simulink model "Base_Map_cs"  (R2019a)
settings: Solver=FixedStepDiscrete  StartTime=0.0  StopTime=15  FixedStep=1/300  RelTol=1e-3
PreLoadFcn:
  | mbxruntime.callbacks.PreLoadFcn(bdroot);
  | check_NUTS_defined
  | model_closed = 0;
  | assignin('base',['model_closed_' bdroot],false);
PostLoadFcn:
  | mbxruntime.callbacks.PostLoadFcn(bdroot);
InitFcn:
  | mbxruntime.callbacks.InitFcn(bdroot);
StartFcn:
  | mbxruntime.callbacks.StartFcn(bdroot);
StopFcn:
  | mbxruntime.callbacks.StopFcn(bdroot);;
  | 
model workspace: external: MAT-File .\Base_Map_S_cs_hws.mat (data not in the file)
undefined symbols (not defined in the file or in its folder): AngularVelocity, Clock_, Data, Data_SL_Info, DiscIntNeverNeededParam, Encoding, Encoding_SL_Info, Header, Height, InitImageOutputDir, LinearAcceleration, mbxruntime, Orientation, Pose, Poses, Poses_SL_Info, Position, Step, tabledata, Twist, Width
libraries: PBCSimulinkLibrary x53, robotlib x26, simulink_extras x19, PreScanSimulinkLibrary x6, dspindex x4, robotcorelib x2, sharedtransform x2, visionconversions x1, visionsinks x1
(part 5 of 8)

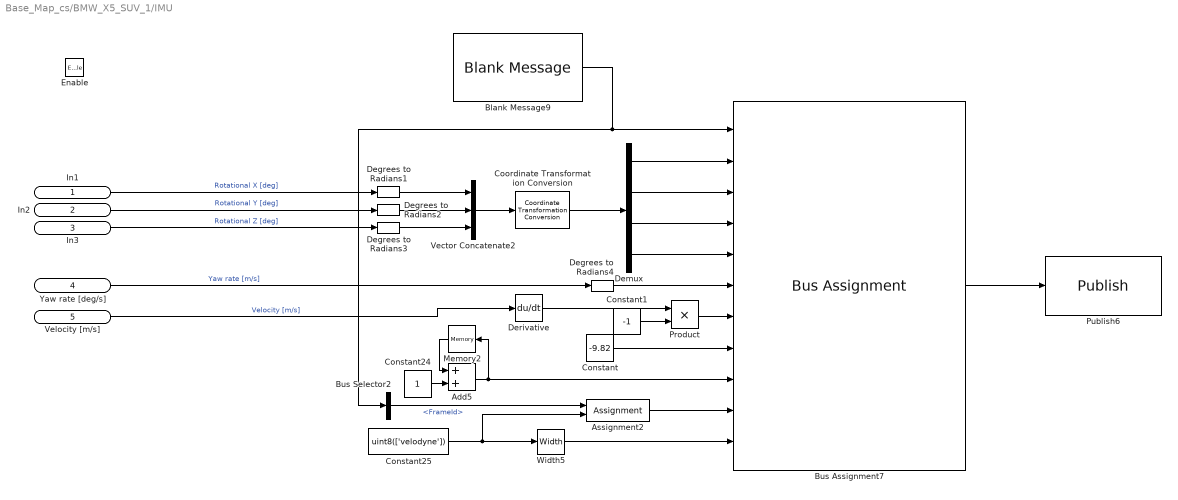
== system Base_Map_cs/BMW_X5_SUV_1/IMU ==
  In1 : Inport
  In2 : Inport  Port=2
  In3 : Inport  Port=3
  Yaw rate [deg/s] : Inport  Port=4
  Velocity [m/s] : Inport  Port=5
  Enable : EnablePort
  Add5 : Sum
  Assignment2 : Assignment  OutputInitialize=Specify size for each dimension in table  DiagnosticForDimensions=Warning  IndexOptions=Starting index (dialog)  Indices=1  OutputSizes=1000
  Blank Message9 : robotlib/Blank Message  messageClass=Message  entityType=sensor_msgs/Imu  messageType=sensor_msgs/Imu  SampleTime=inf
      settings: SourceProductBaseCode=RO
  Bus Assignment7 : BusAssignment  AssignedSignals=Orientation.W,Orientation.X,Orientation.Y,Orientation.Z,AngularVelocity.Z,LinearAcceleration.X,LinearAcceleration.Z,Header.Seq,Header.FrameId,Header.FrameId_SL_Info.CurrentLength
  Bus Selector2 : BusSelector  OutputSignals=Header.FrameId
  Constant : Constant  Value=-9.82
  Constant1 : Constant  Value=-1
  Constant24 : Constant  OutDataTypeStr=uint32
  Constant25 : Constant  Value=uint8(['velodyne'])
  Coordinate Transformation Conversion : robotcorelib/Coordinate Transformation Conversion  InputRepresentation=Euler Angles  InputEulerSequence=XYZ  ShowTrVecInputPort=on  OutputRepresentation=Quaternion  OutputEulerSequence=ZYX  ShowTrVecOutputPort=on  SimulateUsing=Interpreted execution
      settings: SourceProductBaseCode=RO
  Degrees to Radians{1..4} (4 alike) : simulink_extras/Transformations/Degrees to Radians
  Demux : Demux
  Derivative : Derivative
  Memory2 : Memory  InheritSampleTime=on
  Product : Product
  Publish6 : robotlib/Publish  topicSource=Select from ROS network  topic=/imu_raw  messageType=sensor_msgs/Imu  messageQueueLength=1
      settings: SourceProductBaseCode=RO
  Vector Concatenate2 : Concatenate  NumInputs=3
  Width5 : Width  DataType=uint32
  wires:
  Product/1 -> Bus Assignment7/7
  Constant1/1 -> Product/2
  In3/1 -> Degrees to Radians3/1  "Rotational Z [deg]"
  In2/1 -> Degrees to Radians2/1  "Rotational Y [deg]"
  In1/1 -> Degrees to Radians1/1  "Rotational X [deg]"
  Constant/1 -> Bus Assignment7/8
  Velocity [m/s]/1 -> Derivative/1  "Velocity [m/s]"
  Yaw rate [deg/s]/1 -> Degrees to Radians4/1  "Yaw rate [m/s]"
  Demux/4 -> Bus Assignment7/5
  Demux/1 -> Bus Assignment7/2
  Coordinate Transformation Conversion/1 -> Demux/1
  Demux/3 -> Bus Assignment7/4
  Vector Concatenate2/1 -> Coordinate Transformation Conversion/1
  Degrees to Radians3/1 -> Vector Concatenate2/3
  Demux/2 -> Bus Assignment7/3
  Degrees to Radians2/1 -> Vector Concatenate2/2
  Derivative/1 -> Product/1
  Assignment2/1 -> Bus Assignment7/10
  Degrees to Radians4/1 -> Bus Assignment7/6
  Memory2/1 -> Add5/1
  Bus Assignment7/1 -> Publish6/1
  Add5/1 -> Bus Assignment7/9, Memory2/1
  Width5/1 -> Bus Assignment7/11
  Blank Message9/1 -> Bus Assignment7/1, Bus Selector2/1
  Bus Selector2/1 -> Assignment2/1  "<FrameId>"
  Constant25/1 -> Width5/1, Assignment2/2
  Constant24/1 -> Add5/2
  Degrees to Radians1/1 -> Vector Concatenate2/1

== system Base_Map_cs/BMW_X5_SUV_1/PhysicsBasedCameraSensor_1_PBCPose_Control_Mux ==
  Position [m] : Inport
  Orientation [rad] : Inport  Port=2
  Bus Creator1 : BusCreator  Inputs=12  OutDataTypeStr=Bus: PRESCAN_PBCPOSE_DATA  NonVirtualBus=on
  Demux{,1..3} (4 alike) : Demux  Outputs=3
  SignalChanged : PBCSimulinkLibrary/SignalChanged  SystemSampleTime=-1
  SignalChanged1 : PBCSimulinkLibrary/SignalChanged  SystemSampleTime=-1
  Bus : Outport
  wires:
  Demux1/3 -> Bus Creator1/12  "OrientationYaw"
  Demux1/2 -> Bus Creator1/11  "OrientationPitch"
  Demux1/1 -> Bus Creator1/10  "OrientationRoll"
  Demux3/3 -> Bus Creator1/9  "OrientationYawDefined"
  Demux3/2 -> Bus Creator1/8  "OrientationPitchDefined"
  Demux3/1 -> Bus Creator1/7  "OrientationRollDefined"
  Demux/3 -> Bus Creator1/6  "PositionZ"
  Demux/2 -> Bus Creator1/5  "PositionY"
  Demux/1 -> Bus Creator1/4  "PositionX"
  Demux2/3 -> Bus Creator1/3  "PositionZDefined"
  Demux2/2 -> Bus Creator1/2  "PositionYDefined"
  Demux2/1 -> Bus Creator1/1  "PositionXDefined"
  SignalChanged1/1 -> Demux3/1
  SignalChanged/1 -> Demux2/1
  Bus Creator1/1 -> Bus/1
  Position [m]/1 -> SignalChanged/1, Demux/1
  Orientation [rad]/1 -> SignalChanged1/1, Demux1/1

== system Base_Map_cs/BMW_X5_SUV_1/PhysicsBasedCameraSensor_1_PBC_Control_Mux ==
  IntegrationTime [s] : Inport
  DigitalGain [-] : Inport  Port=2
  InterRowIntegrationDelay [s] : Inport  Port=3
  AnalogGain : Constant  Value=0
  AnalogGainDefined : Constant  Value=false
  Bus Creator1 : BusCreator  Inputs=14  OutDataTypeStr=Bus: PRESCAN_PBCCONTROL_DATA  NonVirtualBus=on
  DigitalGain1 : Constant  Value=0
  DigitalGain2 : Constant  Value=0
  DigitalGain3 : Constant  Value=0
  DigitalGainDefined1 : Constant  Value=false
  DigitalGainDefined2 : Constant  Value=false
  DigitalGainDefined3 : Constant  Value=false
  NonNegativeSignalChanged1 : PBCSimulinkLibrary/NonNegativeSignalChanged  SystemSampleTime=-1
  NonNegativeSignalChanged2 : PBCSimulinkLibrary/NonNegativeSignalChanged  SystemSampleTime=-1
  NonNegativeSignalChanged7 : PBCSimulinkLibrary/NonNegativeSignalChanged  SystemSampleTime=-1
  Bus : Outport
  wires:
  NonNegativeSignalChanged7/1 -> Bus Creator1/13  "InterRowIntegrationDelayDefined"
  InterRowIntegrationDelay [s]/1 -> Bus Creator1/14, NonNegativeSignalChanged7/1  "InterRowIntegrationDelay"
  AnalogGainDefined/1 -> Bus Creator1/11  "AnalogGainDefined"
  AnalogGain/1 -> Bus Creator1/12  "AnalogGain"
  DigitalGainDefined3/1 -> Bus Creator1/9  "DigitalGain3Defined"
  DigitalGainDefined2/1 -> Bus Creator1/7  "DigitalGain2Defined"
  DigitalGainDefined1/1 -> Bus Creator1/5  "DigitalGain1Defined"
  NonNegativeSignalChanged2/1 -> Bus Creator1/3  "DigitalGain0Defined"
  NonNegativeSignalChanged1/1 -> Bus Creator1/1  "IntegrationTimeDefined"
  DigitalGain3/1 -> Bus Creator1/10  "DigitalGain3"
  DigitalGain2/1 -> Bus Creator1/8  "DigitalGain2"
  DigitalGain1/1 -> Bus Creator1/6  "DigitalGain1"
  DigitalGain [-]/1 -> Bus Creator1/4, NonNegativeSignalChanged2/1  "DigitalGain0"
  IntegrationTime [s]/1 -> Bus Creator1/2, NonNegativeSignalChanged1/1  "IntegrationTime"
  Bus Creator1/1 -> Bus/1

== system Base_Map_cs/BMW_X5_SUV_1/PhysicsBasedCameraSensor_1_capture_opticsandsensor_Demux ==
  note: This block exists for legacy compatibility only
  In1 : Inport
  I : Outport
  wires:
  In1/1 -> I/1

== system Base_Map_cs/BMW_X5_SUV_1/PointCloudSensor_1_Angles_Demux ==
  In2 : Inport
  Selector : Selector  NumberOfDimensions=2  InputPortWidth=3  IndexOptions=Index vector (dialog),Index vector (dialog)  Indices=-1,offset+1:(offset+hres)  OutputSizes=1,1
  Selector1 : Selector  NumberOfDimensions=2  InputPortWidth=3  IndexOptions=Index vector (dialog),Index vector (dialog)  Indices=-1,(offset+hres+1):(offset+2*hres)  OutputSizes=1,1
  Theta : Outport
  Phi : Outport  Port=2
  wires:
  Selector1/1 -> Phi/1
  Selector/1 -> Theta/1
  In2/1 -> Selector/1, Selector1/1

== system Base_Map_cs/BMW_X5_SUV_1/PointCloudSensor_1_Intensity_Demux ==
  In1 : Inport
  Selector3 : Selector  NumberOfDimensions=2  InputPortWidth=3  IndexOptions=Index vector (dialog),Index vector (dialog)  Indices=-1,offset+1:(offset+hres)  OutputSizes=1,1
  Intensity : Outport
  wires:
  Selector3/1 -> Intensity/1
  In1/1 -> Selector3/1

== system Base_Map_cs/BMW_X5_SUV_1/PointCloudSensor_1_Range_Demux ==
  In1 : Inport
  Selector : Selector  NumberOfDimensions=2  InputPortWidth=3  IndexOptions=Index vector (dialog),Index vector (dialog)  Indices=-1,offset+1:(offset+hres)  OutputSizes=1,1
  Range : Outport
  wires:
  Selector/1 -> Range/1
  In1/1 -> Selector/1

== system Base_Map_cs/BMW_X5_SUV_1/PointCloudSensor_2_Angles_Demux ==
  In2 : Inport
  Selector : Selector  NumberOfDimensions=2  InputPortWidth=3  IndexOptions=Index vector (dialog),Index vector (dialog)  Indices=-1,offset+1:(offset+hres)  OutputSizes=1,1
  Selector1 : Selector  NumberOfDimensions=2  InputPortWidth=3  IndexOptions=Index vector (dialog),Index vector (dialog)  Indices=-1,(offset+hres+1):(offset+2*hres)  OutputSizes=1,1
  Theta : Outport
  Phi : Outport  Port=2
  wires:
  Selector1/1 -> Phi/1
  Selector/1 -> Theta/1
  In2/1 -> Selector/1, Selector1/1

== system Base_Map_cs/BMW_X5_SUV_1/PointCloudSensor_2_Intensity_Demux ==
  In1 : Inport
  Selector3 : Selector  NumberOfDimensions=2  InputPortWidth=3  IndexOptions=Index vector (dialog),Index vector (dialog)  Indices=-1,offset+1:(offset+hres)  OutputSizes=1,1
  Intensity : Outport
  wires:
  Selector3/1 -> Intensity/1
  In1/1 -> Selector3/1

== system Base_Map_cs/BMW_X5_SUV_1/PointCloudSensor_2_Range_Demux ==
  In1 : Inport
  Selector : Selector  NumberOfDimensions=2  InputPortWidth=3  IndexOptions=Index vector (dialog),Index vector (dialog)  Indices=-1,offset+1:(offset+hres)  OutputSizes=1,1
  Range : Outport
  wires:
  Selector/1 -> Range/1
  In1/1 -> Selector/1

== system Base_Map_cs/BMW_X5_SUV_1/PointCloudSensor_3_Angles_Demux ==
  In2 : Inport
  Selector : Selector  NumberOfDimensions=2  InputPortWidth=3  IndexOptions=Index vector (dialog),Index vector (dialog)  Indices=-1,offset+1:(offset+hres)  OutputSizes=1,1
  Selector1 : Selector  NumberOfDimensions=2  InputPortWidth=3  IndexOptions=Index vector (dialog),Index vector (dialog)  Indices=-1,(offset+hres+1):(offset+2*hres)  OutputSizes=1,1
  Theta : Outport
  Phi : Outport  Port=2
  wires:
  Selector1/1 -> Phi/1
  Selector/1 -> Theta/1
  In2/1 -> Selector/1, Selector1/1

== system Base_Map_cs/BMW_X5_SUV_1/PointCloudSensor_3_Intensity_Demux ==
  In1 : Inport
  Selector3 : Selector  NumberOfDimensions=2  InputPortWidth=3  IndexOptions=Index vector (dialog),Index vector (dialog)  Indices=-1,offset+1:(offset+hres)  OutputSizes=1,1
  Intensity : Outport
  wires:
  Selector3/1 -> Intensity/1
  In1/1 -> Selector3/1

== system Base_Map_cs/BMW_X5_SUV_1/PointCloudSensor_3_Range_Demux ==
  In1 : Inport
  Selector : Selector  NumberOfDimensions=2  InputPortWidth=3  IndexOptions=Index vector (dialog),Index vector (dialog)  Indices=-1,offset+1:(offset+hres)  OutputSizes=1,1
  Range : Outport
  wires:
  Selector/1 -> Range/1
  In1/1 -> Selector/1

== system Base_Map_cs/BMW_X5_SUV_1/PointCloudSensor_4_Angles_Demux ==
  In2 : Inport
  Selector : Selector  NumberOfDimensions=2  InputPortWidth=3  IndexOptions=Index vector (dialog),Index vector (dialog)  Indices=-1,offset+1:(offset+hres)  OutputSizes=1,1
  Selector1 : Selector  NumberOfDimensions=2  InputPortWidth=3  IndexOptions=Index vector (dialog),Index vector (dialog)  Indices=-1,(offset+hres+1):(offset+2*hres)  OutputSizes=1,1
  Theta : Outport
  Phi : Outport  Port=2
  wires:
  Selector1/1 -> Phi/1
  Selector/1 -> Theta/1
  In2/1 -> Selector/1, Selector1/1

== system Base_Map_cs/BMW_X5_SUV_1/PointCloudSensor_4_Intensity_Demux ==
  In1 : Inport
  Selector3 : Selector  NumberOfDimensions=2  InputPortWidth=3  IndexOptions=Index vector (dialog),Index vector (dialog)  Indices=-1,offset+1:(offset+hres)  OutputSizes=1,1
  Intensity : Outport
  wires:
  Selector3/1 -> Intensity/1
  In1/1 -> Selector3/1

== system Base_Map_cs/BMW_X5_SUV_1/PointCloudSensor_4_Range_Demux ==
  In1 : Inport
  Selector : Selector  NumberOfDimensions=2  InputPortWidth=3  IndexOptions=Index vector (dialog),Index vector (dialog)  Indices=-1,offset+1:(offset+hres)  OutputSizes=1,1
  Range : Outport
  wires:
  Selector/1 -> Range/1
  In1/1 -> Selector/1

== system Base_Map_cs/BMW_X5_SUV_1/SELF_Demux ==
  SELF : Inport  OutDataTypeStr=Bus: PRESCAN_SELFSENSORDATA
  Bus Selector : BusSelector  OutputSignals=PositionX,PositionY,PositionZ,OrientationRoll,OrientationPitch,OrientationYaw,Velocity,Yaw_rate,Lat,Long,Alt
  Demux2 : Demux  Outputs=3
  Gain : Gain  Gain=180/pi
  Gain1 : Gain  Gain=180/pi
  Vector Concatenate1 : Concatenate  NumInputs=3
  compas converter : Subsystem
  x [m] : Outport
  y [m] : Outport  Port=2
  z [m] : Outport  Port=3
  rotx [deg] : Outport  Port=4
  roty [deg] : Outport  Port=5
  rotz [deg] : Outport  Port=6
  GPS lat [deg] : Outport  Port=7
  GPS long [deg] : Outport  Port=8
  GPS alt [m] : Outport  Port=9
  velocity [m/s] : Outport  Port=10
  heading [deg] : Outport  Port=11
  yaw rate [deg/s] : Outport  Port=12
  wires:
  Bus Selector/11 -> GPS alt [m]/1  "<Alt>"
  Bus Selector/10 -> GPS long [deg]/1  "<Long>"
  Bus Selector/9 -> GPS lat [deg]/1  "<Lat>"
  Bus Selector/8 -> Gain1/1  "<Yaw_rate>"
  Bus Selector/7 -> velocity [m/s]/1  "<Velocity>"
  Bus Selector/6 -> compas converter/1(rotz [rad]), Vector Concatenate1/3  "<OrientationYaw>"
  Bus Selector/5 -> Vector Concatenate1/2  "<OrientationPitch>"
  Bus Selector/4 -> Vector Concatenate1/1  "<OrientationRoll>"
  Vector Concatenate1/1 -> Gain/1
  Bus Selector/3 -> z [m]/1  "<PositionZ>"
  Bus Selector/2 -> y [m]/1  "<PositionY>"
  Bus Selector/1 -> x [m]/1  "<PositionX>"
  SELF/1 -> Bus Selector/1
  Gain/1 -> Demux2/1
  Demux2/1 -> rotx [deg]/1
  Demux2/2 -> roty [deg]/1
  Demux2/3 -> rotz [deg]/1
  compas converter/1(heading [deg]) -> heading [deg]/1
  Gain1/1 -> yaw rate [deg/s]/1

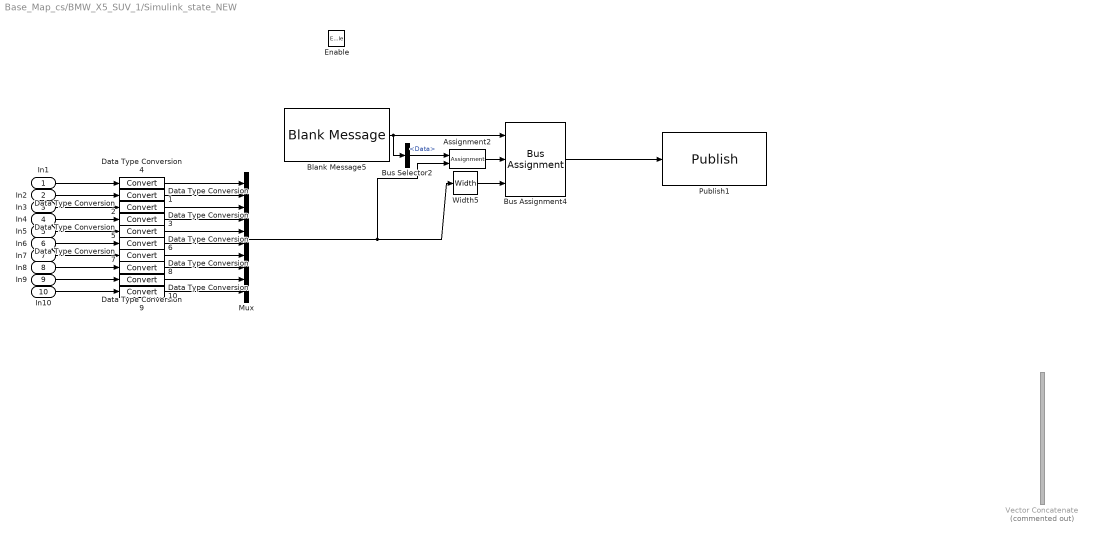
== system Base_Map_cs/BMW_X5_SUV_1/Simulink_state_NEW ==
  In1 : Inport
  In2 : Inport  Port=2
  In3 : Inport  Port=3
  In4 : Inport  Port=4
  In5 : Inport  Port=5
  In6 : Inport  Port=6
  In7 : Inport  Port=7
  In8 : Inport  Port=8
  In9 : Inport  Port=9
  In10 : Inport  Port=10
  Enable : EnablePort
  Assignment2 : Assignment  OutputInitialize=Specify size for each dimension in table  DiagnosticForDimensions=Warning  IndexOptions=Starting index (dialog)  Indices=1  OutputSizes=1000
  Blank Message5 : robotlib/Blank Message  messageClass=Message  entityType=std_msgs/Int32MultiArray  messageType=std_msgs/Int32MultiArray  SampleTime=inf
      settings: SourceProductBaseCode=RO
  Bus Assignment4 : BusAssignment  AssignedSignals=Data,Data_SL_Info.CurrentLength
  Bus Selector2 : BusSelector  OutputSignals=Data
  Data Type Conversion{1..10} (10 alike) : DataTypeConversion
  Mux : Mux  Inputs=10
  Publish1 : robotlib/Publish  topicSource=Specify your own  topic=/Simulink_state  messageType=std_msgs/Int32MultiArray  messageQueueLength=1
      settings: SourceProductBaseCode=RO
  Vector Concatenate : Concatenate  Commented=on  NumInputs=10
  Width5 : Width  DataType=uint32
  wires:
  Assignment2/1 -> Bus Assignment4/2
  Blank Message5/1 -> Bus Assignment4/1, Bus Selector2/1
  Bus Selector2/1 -> Assignment2/1  "<Data>"
  In7/1 -> Data Type Conversion7/1
  In10/1 -> Data Type Conversion10/1
  In9/1 -> Data Type Conversion9/1
  In8/1 -> Data Type Conversion8/1
  In6/1 -> Data Type Conversion6/1
  In5/1 -> Data Type Conversion5/1
  In4/1 -> Data Type Conversion3/1
  In3/1 -> Data Type Conversion2/1
  In2/1 -> Data Type Conversion1/1
  Data Type Conversion10/1 -> Mux/10
  Data Type Conversion9/1 -> Mux/9
  Data Type Conversion8/1 -> Mux/8
  Data Type Conversion7/1 -> Mux/7
  Data Type Conversion6/1 -> Mux/6
  Data Type Conversion5/1 -> Mux/5
  Data Type Conversion3/1 -> Mux/4
  Data Type Conversion2/1 -> Mux/3
  Data Type Conversion1/1 -> Mux/2
  Width5/1 -> Bus Assignment4/3
  Mux/1 -> Width5/1, Assignment2/2
  Bus Assignment4/1 -> Publish1/1
  Data Type Conversion4/1 -> Mux/1
  In1/1 -> Data Type Conversion4/1

== system Base_Map_cs/BMW_X5_SUV_1/Subsystem ==
  In1 : Inport
  In2 : Inport  Port=2
  In3 : Inport  Port=3
  In4 : Inport  Port=4
  In5 : Inport  Port=5
  Matrix Concatenate5 : Concatenate  NumInputs=4  Mode=Multidimensional array  ConcatenateDimension=2
  Reshape{1..4} (4 alike) : Reshape
  Rotate over Z : Subsystem
  Spherical to cartesian : Subsystem
  Out1 : Outport
  wires:
  In4/1 -> Reshape2/1
  In2/1 -> Reshape4/1
  Matrix Concatenate5/1 -> Out1/1
  Rotate over Z/1(Out1) -> Matrix Concatenate5/1
  Reshape3/1 -> Matrix Concatenate5/4
  Spherical to cartesian/3(Out3) -> Matrix Concatenate5/3
  Rotate over Z/2(Out2) -> Matrix Concatenate5/2
  In3/1 -> Reshape1/1
  Spherical to cartesian/2(Out2) -> Rotate over Z/3(In3)
  Reshape2/1 -> Spherical to cartesian/3(In3)
  Spherical to cartesian/1(Out1) -> Rotate over Z/2(In2)
  Reshape1/1 -> Spherical to cartesian/2(In2)
  In1/1 -> Rotate over Z/1(In1)
  Reshape4/1 -> Spherical to cartesian/1(In1)
  In5/1 -> Reshape3/1

== system Base_Map_cs/BMW_X5_SUV_1/Subsystem1 ==
  In1 : Inport
  In2 : Inport  Port=2
  In3 : Inport  Port=3
  In4 : Inport  Port=4
  In5 : Inport  Port=5
  Matrix Concatenate5 : Concatenate  NumInputs=4  Mode=Multidimensional array  ConcatenateDimension=2
  Reshape{1..4} (4 alike) : Reshape
  Rotate over Z : Subsystem
  Spherical to cartesian : Subsystem
  Out1 : Outport
  wires:
  In4/1 -> Reshape2/1
  In2/1 -> Reshape4/1
  Matrix Concatenate5/1 -> Out1/1
  Rotate over Z/1(Out1) -> Matrix Concatenate5/1
  Reshape3/1 -> Matrix Concatenate5/4
  Spherical to cartesian/3(Out3) -> Matrix Concatenate5/3
  Rotate over Z/2(Out2) -> Matrix Concatenate5/2
  In3/1 -> Reshape1/1
  Spherical to cartesian/2(Out2) -> Rotate over Z/3(In3)
  Reshape2/1 -> Spherical to cartesian/3(In3)
  Spherical to cartesian/1(Out1) -> Rotate over Z/2(In2)
  Reshape1/1 -> Spherical to cartesian/2(In2)
  In1/1 -> Rotate over Z/1(In1)
  Reshape4/1 -> Spherical to cartesian/1(In1)
  In5/1 -> Reshape3/1

== system Base_Map_cs/BMW_X5_SUV_1/Subsystem2 ==
  In1 : Inport
  In2 : Inport  Port=2
  In3 : Inport  Port=3
  In4 : Inport  Port=4
  In5 : Inport  Port=5
  Matrix Concatenate5 : Concatenate  NumInputs=4  Mode=Multidimensional array  ConcatenateDimension=2
  Reshape{1..4} (4 alike) : Reshape
  Rotate over Z : Subsystem
  Spherical to cartesian : Subsystem
  Out1 : Outport
  wires:
  In4/1 -> Reshape2/1
  In2/1 -> Reshape4/1
  Matrix Concatenate5/1 -> Out1/1
  Rotate over Z/1(Out1) -> Matrix Concatenate5/1
  Reshape3/1 -> Matrix Concatenate5/4
  Spherical to cartesian/3(Out3) -> Matrix Concatenate5/3
  Rotate over Z/2(Out2) -> Matrix Concatenate5/2
  In3/1 -> Reshape1/1
  Spherical to cartesian/2(Out2) -> Rotate over Z/3(In3)
  Reshape2/1 -> Spherical to cartesian/3(In3)
  Spherical to cartesian/1(Out1) -> Rotate over Z/2(In2)
  Reshape1/1 -> Spherical to cartesian/2(In2)
  In1/1 -> Rotate over Z/1(In1)
  Reshape4/1 -> Spherical to cartesian/1(In1)
  In5/1 -> Reshape3/1

== system Base_Map_cs/BMW_X5_SUV_1/Subsystem3 ==
  In1 : Inport
  In2 : Inport  Port=2
  In3 : Inport  Port=3
  In4 : Inport  Port=4
  In5 : Inport  Port=5
  Matrix Concatenate5 : Concatenate  NumInputs=4  Mode=Multidimensional array  ConcatenateDimension=2
  Reshape{1..4} (4 alike) : Reshape
  Rotate over Z : Subsystem
  Spherical to cartesian : Subsystem
  Out1 : Outport
  wires:
  In4/1 -> Reshape2/1
  In2/1 -> Reshape4/1
  Matrix Concatenate5/1 -> Out1/1
  Rotate over Z/1(Out1) -> Matrix Concatenate5/1
  Reshape3/1 -> Matrix Concatenate5/4
  Spherical to cartesian/3(Out3) -> Matrix Concatenate5/3
  Rotate over Z/2(Out2) -> Matrix Concatenate5/2
  In3/1 -> Reshape1/1
  Spherical to cartesian/2(Out2) -> Rotate over Z/3(In3)
  Reshape2/1 -> Spherical to cartesian/3(In3)
  Spherical to cartesian/1(Out1) -> Rotate over Z/2(In2)
  Reshape1/1 -> Spherical to cartesian/2(In2)
  In1/1 -> Rotate over Z/1(In1)
  Reshape4/1 -> Spherical to cartesian/1(In1)
  In5/1 -> Reshape3/1

== system Base_Map_cs/BMW_X5_SUV_1/Subsystem4 ==
  Enable : EnablePort
  Bus Selector : BusSelector  OutputSignals=Pose.Position.X
  Subscribe : robotlib/Subscribe  topicSource=Specify your own  topic=/current_pose  messageType=geometry_msgs/PoseStamped  sampleTime=-1  messageQueueLength=1
      settings: SourceProductBaseCode=RO
  Terminator_6 : Terminator
  To Workspace : ToWorkspace  VariableName=Values_of_X  SaveFormat=Timeseries  SampleTime=-1
  wires:
  Subscribe/1 -> Terminator_6/1
  Subscribe/2 -> Bus Selector/1
  Bus Selector/1 -> To Workspace/1  "<X>"

== system Base_Map_cs/BMW_X5_SUV_1/camera_CM_Demux ==
  In1 : Inport
  Selector : Selector  NumberOfDimensions=2  InputPortWidth=3  IndexOptions=Index vector (dialog),Index vector (dialog)  Indices=-1,1:hres  OutputSizes=1,1
  Selector1 : Selector  NumberOfDimensions=2  InputPortWidth=3  IndexOptions=Index vector (dialog),Index vector (dialog)  Indices=-1,hres+1:hres*2  OutputSizes=1,1
  Selector2 : Selector  NumberOfDimensions=2  InputPortWidth=3  IndexOptions=Index vector (dialog),Index vector (dialog)  Indices=-1,hres*2+1:hres*3  OutputSizes=1,1
  R : Outport
  G : Outport  Port=2
  B : Outport  Port=3
  wires:
  In1/1 -> Selector1/1, Selector/1, Selector2/1
  Selector/1 -> R/1
  Selector1/1 -> G/1
  Selector2/1 -> B/1

== system Base_Map_cs/BMW_X5_SUV_1/clock ==
  note: Nanoseconds
  In1 : Inport
  Enable : EnablePort
  Blank Message3 : robotlib/Blank Message  messageClass=Message  entityType=rosgraph_msgs/Clock  messageType=rosgraph_msgs/Clock  SampleTime=inf
      settings: SourceProductBaseCode=RO
  Bus Assignment : BusAssignment  AssignedSignals=Clock_.Sec,Clock_.Nsec
  Constant2 : Constant  Value=1000000000
  Floor : Rounding  Operator=fix
  Product : Product
  Publish3 : robotlib/Publish  topicSource=Specify your own  topic=/clock  messageType=rosgraph_msgs/Clock  messageQueueLength=1
      settings: SourceProductBaseCode=RO
  Subtract : Sum  Inputs=+-
  wires:
  In1/1 -> Subtract/1, Floor/1
  Floor/1 -> Subtract/2, Bus Assignment/2
  Blank Message3/1 -> Bus Assignment/1
  Bus Assignment/1 -> Publish3/1
  Subtract/1 -> Product/1
  Product/1 -> Bus Assignment/3
  Constant2/1 -> Product/2

== system Base_Map_cs/BMW_X5_SUV_1/current_velocity ==
  In1 : Inport
  In2 : Inport  Port=2
  Enable : EnablePort
  Add5 : Sum
  Assignment2 : Assignment  OutputInitialize=Specify size for each dimension in table  DiagnosticForDimensions=Warning  IndexOptions=Starting index (dialog)  Indices=1  OutputSizes=1000
  Blank Message6 : robotlib/Blank Message  messageClass=Message  entityType=geometry_msgs/TwistStamped  messageType=geometry_msgs/TwistStamped  SampleTime=inf
      settings: SourceProductBaseCode=RO
  Bus Assignment5 : BusAssignment  AssignedSignals=Header.Seq,Header.FrameId,Header.FrameId_SL_Info.CurrentLength,Twist.Linear.X,Twist.Linear.Y,Twist.Linear.Z,Twist.Angular.X,Twist.Angular.Y,Twist.Angular.Z
  Bus Selector2 : BusSelector  OutputSignals=Header.FrameId
  Constant{18..21} (4 alike) : Constant  Value=0
  Constant24 : Constant  OutDataTypeStr=uint32
  Constant25 : Constant  Value=uint8(['/base_link'])
  Degrees to Radians3 : simulink_extras/Transformations/Degrees to Radians
  Memory2 : Memory  InheritSampleTime=on
  Publish4 : robotlib/Publish  topicSource=Select from ROS network  topic=/current_velocity  messageType=geometry_msgs/TwistStamped  messageQueueLength=1
      settings: SourceProductBaseCode=RO
  Width5 : Width  DataType=uint32
  wires:
  Constant25/1 -> Assignment2/2, Width5/1
  Assignment2/1 -> Bus Assignment5/3
  Memory2/1 -> Add5/1
  Degrees to Radians3/1 -> Bus Assignment5/10
  Constant19/1 -> Bus Assignment5/7
  Constant24/1 -> Add5/2
  Width5/1 -> Bus Assignment5/4
  Constant20/1 -> Bus Assignment5/8
  Bus Selector2/1 -> Assignment2/1  "<FrameId>"
  Add5/1 -> Bus Assignment5/2, Memory2/1
  Constant18/1 -> Bus Assignment5/6
  Blank Message6/1 -> Bus Selector2/1, Bus Assignment5/1
  Constant21/1 -> Bus Assignment5/9
  Bus Assignment5/1 -> Publish4/1
  In1/1 -> Bus Assignment5/5
  In2/1 -> Degrees to Radians3/1

== system Base_Map_cs/BMW_X5_SUV_1/gnss_pose_simulink ==
  In1 : Inport
  Enable : EnablePort
  Blank Message4 : robotlib/Blank Message  messageClass=Message  entityType=geometry_msgs/Pose  messageType=geometry_msgs/Pose  SampleTime=inf
      settings: SourceProductBaseCode=RO
  Bus Assignment3 : BusAssignment  AssignedSignals=Position.X,Position.Y,Position.Z,Orientation.W,Orientation.X,Orientation.Y,Orientation.Z
  Demux : Demux  Outputs=7
  Publish2 : robotlib/Publish  topicSource=Specify your own  topic=/gnss_pose_simulink  messageType=geometry_msgs/Pose  messageQueueLength=1
      settings: SourceProductBaseCode=RO
  wires:
  Bus Assignment3/1 -> Publish2/1
  Blank Message4/1 -> Bus Assignment3/1
  Demux/4 -> Bus Assignment3/5
  Demux/3 -> Bus Assignment3/4
  Demux/5 -> Bus Assignment3/6
  Demux/7 -> Bus Assignment3/8
  Demux/2 -> Bus Assignment3/3
  In1/1 -> Demux/1
  Demux/6 -> Bus Assignment3/7
  Demux/1 -> Bus Assignment3/2

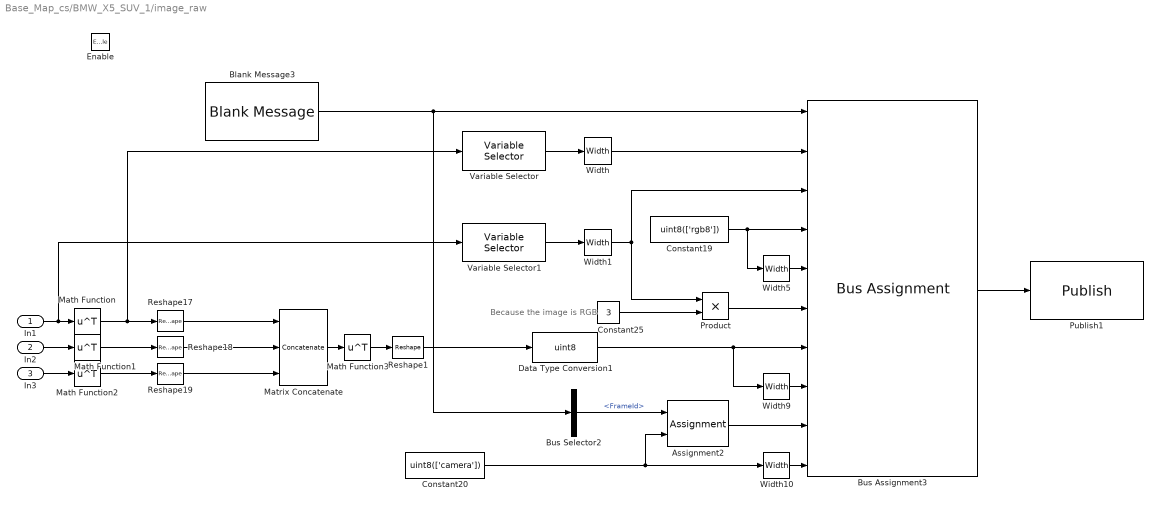
== system Base_Map_cs/BMW_X5_SUV_1/image_raw ==
  note: Because the image is RGB
  In1 : Inport
  In2 : Inport  Port=2
  In3 : Inport  Port=3
  Enable : EnablePort
  Assignment2 : Assignment  OutputInitialize=Specify size for each dimension in table  DiagnosticForDimensions=Warning  IndexOptions=Starting index (dialog)  Indices=1  OutputSizes=1000
  Blank Message3 : robotlib/Blank Message  messageClass=Message  entityType=sensor_msgs/Image  messageType=sensor_msgs/Image  SampleTime=inf
      settings: SourceProductBaseCode=RO
  Bus Assignment3 : BusAssignment  AssignedSignals=Height,Width,Encoding,Encoding_SL_Info.CurrentLength,Step,Data,Data_SL_Info.CurrentLength,Header.FrameId,Header.FrameId_SL_Info.CurrentLength
  Bus Selector2 : BusSelector  OutputSignals=Header.FrameId
  Constant19 : Constant  Value=uint8(['rgb8'])
  Constant20 : Constant  Value=uint8(['camera'])
  Constant25 : Constant  Value=3  OutDataTypeStr=Inherit: Inherit via back propagation
  Data Type Conversion1 : DataTypeConversion  OutDataTypeStr=uint8
  Math Function{,1..3} (4 alike) : Math  Operator=transpose  SaturateOnIntegerOverflow=on
  Matrix Concatenate : Concatenate  NumInputs=3  Mode=Multidimensional array  ConcatenateDimension=2
  Product : Product  OutDataTypeStr=uint32
  Publish1 : robotlib/Publish  topicSource=Specify your own  topic=/image_raw  messageType=sensor_msgs/Image  messageQueueLength=1
      settings: SourceProductBaseCode=RO
  Reshape{1,17..19} (4 alike) : Reshape
  Variable Selector : dspindex/Variable Selector  NumInputs=1  rowsOrCols=Rows  IdxMode=Fixed  Elements=[1]  ZerOneIdxMode=One-based  errmode=Clip Index  FillMode=on  FillValues=0
  Variable Selector1 : dspindex/Variable Selector  NumInputs=1  rowsOrCols=Rows  IdxMode=Fixed  Elements=[1]  ZerOneIdxMode=One-based  errmode=Clip Index  FillMode=on  FillValues=0
  Width : Width
  Width1 : Width
  Width10 : Width  DataType=uint32
  Width5 : Width  DataType=uint32
  Width9 : Width  DataType=uint32
  wires:
  Reshape19/1 -> Matrix Concatenate/3
  Data Type Conversion1/1 -> Width9/1, Bus Assignment3/7
  Math Function/1 -> Variable Selector/1, Reshape17/1
  Constant25/1 -> Product/2
  Width/1 -> Bus Assignment3/2
  Width9/1 -> Bus Assignment3/8
  Bus Selector2/1 -> Assignment2/1  "<FrameId>"
  Product/1 -> Bus Assignment3/6
  Assignment2/1 -> Bus Assignment3/9
  Bus Assignment3/1 -> Publish1/1
  Constant19/1 -> Width5/1, Bus Assignment3/4
  Reshape18/1 -> Matrix Concatenate/2
  Width5/1 -> Bus Assignment3/5
  Reshape17/1 -> Matrix Concatenate/1
  Width10/1 -> Bus Assignment3/10
  Math Function2/1 -> Reshape19/1
  Constant20/1 -> Assignment2/2, Width10/1
  Width1/1 -> Bus Assignment3/3, Product/1
  Math Function1/1 -> Reshape18/1
  Blank Message3/1 -> Bus Selector2/1, Bus Assignment3/1
  In3/1 -> Math Function2/1
  In2/1 -> Math Function1/1
  In1/1 -> Variable Selector1/1, Math Function/1
  Reshape1/1 -> Data Type Conversion1/1
  Matrix Concatenate/1 -> Math Function3/1
  Math Function3/1 -> Reshape1/1
  Variable Selector/1 -> Width/1
  Variable Selector1/1 -> Width1/1

== system Base_Map_cs/BMW_X5_SUV_1/move_base_simple//goal ==
  In1 : Inport
  Enable : EnablePort
  Add4 : Sum
  Assignment4 : Assignment  OutputInitialize=Specify size for each dimension in table  DiagnosticForDimensions=Warning  IndexOptions=Starting index (dialog)  Indices=1  OutputSizes=1000
  Blank Message5 : robotlib/Blank Message  messageClass=Message  entityType=geometry_msgs/PoseStamped  messageType=geometry_msgs/PoseStamped  SampleTime=inf
      settings: SourceProductBaseCode=RO
  Bus Assignment4 : BusAssignment  AssignedSignals=Header.Seq,Header.FrameId,Header.FrameId_SL_Info.CurrentLength,Pose.Position.X,Pose.Position.Y,Pose.Position.Z,Pose.Orientation.W,Pose.Orientation.X,Pose.Orientation.Y,Pose.Orientation.Z
  Bus Selector3 : BusSelector  OutputSignals=Header.FrameId
  Constant8 : Constant  OutDataTypeStr=uint32
  Constant9 : Constant  Value=uint8(['world'])
  Demux : Demux  Outputs=7
  Memory1 : Memory  InheritSampleTime=on
  Publish1 : robotlib/Publish  topicSource=Select from ROS network  topic=/move_base_simple/goal  messageType=geometry_msgs/PoseStamped  messageQueueLength=1
      settings: SourceProductBaseCode=RO
  Width4 : Width  DataType=uint32
  wires:
  Blank Message5/1 -> Bus Selector3/1, Bus Assignment4/1
  Add4/1 -> Bus Assignment4/2, Memory1/1
  Assignment4/1 -> Bus Assignment4/3
  Bus Selector3/1 -> Assignment4/1  "<FrameId>"
  Bus Assignment4/1 -> Publish1/1
  Constant8/1 -> Add4/2
  Constant9/1 -> Assignment4/2, Width4/1
  Memory1/1 -> Add4/1
  Width4/1 -> Bus Assignment4/4
  In1/1 -> Demux/1
  Demux/1 -> Bus Assignment4/5
  Demux/2 -> Bus Assignment4/6
  Demux/3 -> Bus Assignment4/7
  Demux/4 -> Bus Assignment4/8
  Demux/5 -> Bus Assignment4/9
  Demux/6 -> Bus Assignment4/10
  Demux/7 -> Bus Assignment4/11

== system Base_Map_cs/BMW_X5_SUV_1/points_raw_float32 ==
  In1 : Inport
  In5 : Inport  Port=2
  In9 : Inport  Port=3
  In13 : Inport  Port=4
  Enable : EnablePort
  Blank Message3 : robotlib/Blank Message  messageClass=Message  entityType=std_msgs/Float32MultiArray  messageType=std_msgs/Float32MultiArray  SampleTime=inf
      settings: SourceProductBaseCode=RO
  Bus Assignment3 : BusAssignment  AssignedSignals=Data,Data_SL_Info.CurrentLength
  Data Type Conversion2 : DataTypeConversion  OutDataTypeStr=single
  Math Function1 : Math  Operator=transpose  SaturateOnIntegerOverflow=on
  Matrix Concatenate5 : Concatenate  NumInputs=4  Mode=Multidimensional array
  Publish1 : robotlib/Publish  topicSource=Specify your own  topic=/points_raw_float32  messageType=std_msgs/Float32MultiArray  messageQueueLength=1
      settings: SourceProductBaseCode=RO
  Reshape17 : Reshape
  Width5 : Width  DataType=uint32
  wires:
  In13/1 -> Matrix Concatenate5/4
  In9/1 -> Matrix Concatenate5/3
  In5/1 -> Matrix Concatenate5/2
  In1/1 -> Matrix Concatenate5/1
  Math Function1/1 -> Reshape17/1
  Data Type Conversion2/1 -> Bus Assignment3/2, Width5/1
  Blank Message3/1 -> Bus Assignment3/1
  Bus Assignment3/1 -> Publish1/1
  Reshape17/1 -> Data Type Conversion2/1
  Matrix Concatenate5/1 -> Math Function1/1
  Width5/1 -> Bus Assignment3/3

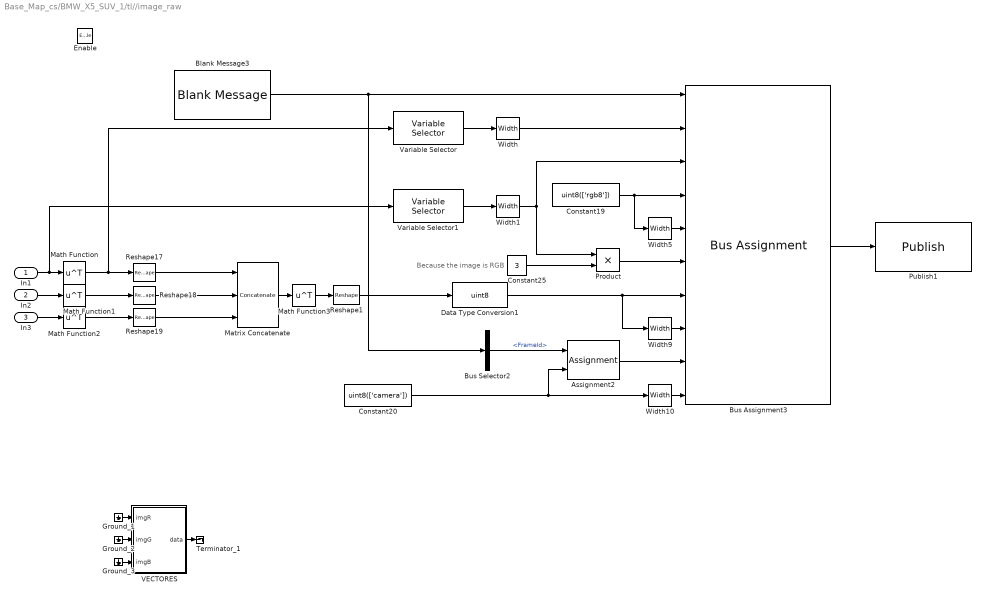
== system Base_Map_cs/BMW_X5_SUV_1/tl//image_raw ==
  note: Because the image is RGB
  In1 : Inport
  In2 : Inport  Port=2
  In3 : Inport  Port=3
  Enable : EnablePort
  Assignment2 : Assignment  OutputInitialize=Specify size for each dimension in table  DiagnosticForDimensions=Warning  IndexOptions=Starting index (dialog)  Indices=1  OutputSizes=1000
  Blank Message3 : robotlib/Blank Message  messageClass=Message  entityType=sensor_msgs/Image  messageType=sensor_msgs/Image  SampleTime=inf
      settings: SourceProductBaseCode=RO
  Bus Assignment3 : BusAssignment  AssignedSignals=Height,Width,Encoding,Encoding_SL_Info.CurrentLength,Step,Data,Data_SL_Info.CurrentLength,Header.FrameId,Header.FrameId_SL_Info.CurrentLength
  Bus Selector2 : BusSelector  OutputSignals=Header.FrameId
  Constant19 : Constant  Value=uint8(['rgb8'])
  Constant20 : Constant  Value=uint8(['camera'])
  Constant25 : Constant  Value=3  OutDataTypeStr=Inherit: Inherit via back propagation
  Data Type Conversion1 : DataTypeConversion  OutDataTypeStr=uint8
  Ground_1 : Ground
  Ground_2 : Ground
  Ground_3 : Ground
  Math Function{,1..3} (4 alike) : Math  Operator=transpose  SaturateOnIntegerOverflow=on
  Matrix Concatenate : Concatenate  NumInputs=3  Mode=Multidimensional array  ConcatenateDimension=2
  Product : Product  OutDataTypeStr=uint32
  Publish1 : robotlib/Publish  topicSource=Specify your own  topic=/tl/image_raw  messageType=sensor_msgs/Image  messageQueueLength=1
      settings: SourceProductBaseCode=RO
  Reshape{1,17..19} (4 alike) : Reshape
  Terminator_1 : Terminator
  VECTORES : MATLAB Function  TreatAsAtomicUnit=on
  Variable Selector : dspindex/Variable Selector  NumInputs=1  rowsOrCols=Rows  IdxMode=Fixed  Elements=[1]  ZerOneIdxMode=One-based  errmode=Clip Index  FillMode=on  FillValues=0
  Variable Selector1 : dspindex/Variable Selector  NumInputs=1  rowsOrCols=Rows  IdxMode=Fixed  Elements=[1]  ZerOneIdxMode=One-based  errmode=Clip Index  FillMode=on  FillValues=0
  Width : Width
  Width1 : Width
  Width10 : Width  DataType=uint32
  Width5 : Width  DataType=uint32
  Width9 : Width  DataType=uint32
  wires:
  Reshape19/1 -> Matrix Concatenate/3
  Data Type Conversion1/1 -> Width9/1, Bus Assignment3/7
  Math Function/1 -> Variable Selector/1, Reshape17/1
  Constant25/1 -> Product/2
  Width/1 -> Bus Assignment3/2
  Width9/1 -> Bus Assignment3/8
  Bus Selector2/1 -> Assignment2/1  "<FrameId>"
  Product/1 -> Bus Assignment3/6
  Assignment2/1 -> Bus Assignment3/9
  Bus Assignment3/1 -> Publish1/1
  Constant19/1 -> Width5/1, Bus Assignment3/4
  Reshape18/1 -> Matrix Concatenate/2
  Width5/1 -> Bus Assignment3/5
  Reshape17/1 -> Matrix Concatenate/1
  Width10/1 -> Bus Assignment3/10
  Math Function2/1 -> Reshape19/1
  Constant20/1 -> Assignment2/2, Width10/1
  Width1/1 -> Bus Assignment3/3, Product/1
  Math Function1/1 -> Reshape18/1
  Blank Message3/1 -> Bus Selector2/1, Bus Assignment3/1
  In3/1 -> Math Function2/1
  In2/1 -> Math Function1/1
  In1/1 -> Variable Selector1/1, Math Function/1
  Reshape1/1 -> Data Type Conversion1/1
  Matrix Concatenate/1 -> Math Function3/1
  Math Function3/1 -> Reshape1/1
  Variable Selector/1 -> Width/1
  Variable Selector1/1 -> Width1/1
  Ground_1/1 -> VECTORES/1(imgR)
  Ground_2/1 -> VECTORES/2(imgG)
  Ground_3/1 -> VECTORES/3(imgB)
  VECTORES/1(data) -> Terminator_1/1

== system Base_Map_cs/BMW_X5_SUV_1/tl_camera_CM_Demux ==
  In1 : Inport
  Selector : Selector  NumberOfDimensions=2  InputPortWidth=3  IndexOptions=Index vector (dialog),Index vector (dialog)  Indices=-1,1:hres  OutputSizes=1,1
  Selector1 : Selector  NumberOfDimensions=2  InputPortWidth=3  IndexOptions=Index vector (dialog),Index vector (dialog)  Indices=-1,hres+1:hres*2  OutputSizes=1,1
  Selector2 : Selector  NumberOfDimensions=2  InputPortWidth=3  IndexOptions=Index vector (dialog),Index vector (dialog)  Indices=-1,hres*2+1:hres*3  OutputSizes=1,1
  R : Outport
  G : Outport  Port=2
  B : Outport  Port=3
  wires:
  In1/1 -> Selector1/1, Selector/1, Selector2/1
  Selector/1 -> R/1
  Selector1/1 -> G/1
  Selector2/1 -> B/1

== system Base_Map_cs/BMW_X5_SUV_1/tonemap ==
  In1 : Inport
  Constant : Constant  Value=255
  Data Type Conversion : DataTypeConversion  OutDataTypeStr=uint8
  Product : Product
  Square Root : Sqrt  SaturateOnIntegerOverflow=on
  Out1 : Outport
  wires:
  Data Type Conversion/1 -> Out1/1
  Constant/1 -> Product/2
  Product/1 -> Data Type Conversion/1
  Square Root/1 -> Product/1
  In1/1 -> Square Root/1

== system Base_Map_cs/BMW_X5_SUV_1/vehicle//odom ==
  In1 : Inport
  In2 : Inport  Port=2
  In3 : Inport  Port=3
  Enable : EnablePort
  Add5 : Sum
  Assignment2 : Assignment  OutputInitialize=Specify size for each dimension in table  DiagnosticForDimensions=Warning  IndexOptions=Starting index (dialog)  Indices=1  OutputSizes=1000
  Blank Message6 : robotlib/Blank Message  messageClass=Message  entityType=nav_msgs/Odometry  messageType=nav_msgs/Odometry  SampleTime=inf
      settings: SourceProductBaseCode=RO
  Bus Assignment5 : BusAssignment  AssignedSignals=Header.Seq,Header.FrameId,Header.FrameId_SL_Info.CurrentLength,ChildFrameId,ChildFrameId_SL_Info.CurrentLength,Pose.Pose.Position.X,Pose.Pose.Position.Y,Pose.Pose.Position.Z,Pose.Pose.Orientation.W,Pose.Pose.Orientation.X,Pose.Pose.Orientation.Y,Pose.Pose.Orientation.Z,Twist.Twist.Linear.X,Twist.Twist.Linear.Y,Twist.Twist.Linear.Z,Twist.Twist.Angular.X,Twist.Twist.Angular.Y,Twist.Twist.Angular.Z
  Bus Selector2 : BusSelector  OutputSignals=Header.FrameId
  Constant{18..21} (4 alike) : Constant  Value=0
  Constant24 : Constant  OutDataTypeStr=uint32
  Constant25 : Constant  Value=uint8(['/base_link'])
  Degrees to Radians3 : simulink_extras/Transformations/Degrees to Radians
  Demux : Demux  Outputs=7
  Memory2 : Memory  InheritSampleTime=on
  Publish4 : robotlib/Publish  topicSource=Specify your own  topic=/vehicle/odom  messageType=nav_msgs/Odometry  messageQueueLength=1
      settings: SourceProductBaseCode=RO
  Width5 : Width  DataType=uint32
  wires:
  Constant25/1 -> Assignment2/2, Width5/1
  Assignment2/1 -> Bus Assignment5/5, Bus Assignment5/3
  Memory2/1 -> Add5/1
  Constant24/1 -> Add5/2
  Width5/1 -> Bus Assignment5/6, Bus Assignment5/4
  Bus Selector2/1 -> Assignment2/1  "<FrameId>"
  Add5/1 -> Bus Assignment5/2, Memory2/1
  Blank Message6/1 -> Bus Selector2/1, Bus Assignment5/1
  Bus Assignment5/1 -> Publish4/1
  In3/1 -> Degrees to Radians3/1
  Constant18/1 -> Bus Assignment5/15
  Degrees to Radians3/1 -> Bus Assignment5/19
  Constant20/1 -> Bus Assignment5/17
  Constant19/1 -> Bus Assignment5/16
  Constant21/1 -> Bus Assignment5/18
  In2/1 -> Bus Assignment5/14
  Demux/3 -> Bus Assignment5/9
  Demux/2 -> Bus Assignment5/8
  Demux/7 -> Bus Assignment5/13
  Demux/6 -> Bus Assignment5/12
  In1/1 -> Demux/1
  Demux/4 -> Bus Assignment5/10
  Demux/5 -> Bus Assignment5/11
  Demux/1 -> Bus Assignment5/7

== system Base_Map_cs/Citroen_C3_Hatchback_1/AIR_2_Demux ==
  AIR : Inport
  Activate_Switch : Subsystem
      mask Display: text(5,10,'')
  Bus Selector : BusSelector  OutputSignals=DATA.Range,DATA.Azimuth,DATA.Elevation,DATA.ID,DATA.Velocity,DATA.Heading
  Data Type Conversion : DataTypeConversion  OutDataTypeStr=double
  For Iterator : ForIterator  ResetStates=reset  IterationLimit=detectableObjects
  Selector : Selector  InputPortWidth=detectableObjects  IndexOptions=Index vector (port)  Indices=[1 3]  OutputSizes=1
  Signal2ArrayOfSignals1 : Subsystem  mask{VECTORLENGTH=detectableObjects}
      mask prompts: VECTORLENGTH "Length of vector"
  Signal2ArrayOfSignals2 : Subsystem  mask{VECTORLENGTH=detectableObjects}
      mask prompts: VECTORLENGTH "Length of vector"
  Signal2ArrayOfSignals3 : Subsystem  mask{VECTORLENGTH=detectableObjects}
      mask prompts: VECTORLENGTH "Length of vector"
  Signal2ArrayOfSignals4 : Subsystem  mask{VECTORLENGTH=detectableObjects}
      mask prompts: VECTORLENGTH "Length of vector"
  Signal2ArrayOfSignals5 : Subsystem  mask{VECTORLENGTH=detectableObjects}
      mask prompts: VECTORLENGTH "Length of vector"
  Signal2ArrayOfSignals6 : Subsystem  mask{VECTORLENGTH=detectableObjects}
      mask prompts: VECTORLENGTH "Length of vector"
  Range [m] : Outport
  Azimuth [deg] : Outport  Port=2
  Elevation [deg] : Outport  Port=3
  ID [-] : Outport  Port=4
  Velocity [m/s] : Outport  Port=5
  Heading [deg] : Outport  Port=6
  wires:
  Data Type Conversion/1 -> ID [-]/1
  Bus Selector/6 -> Signal2ArrayOfSignals6/2(Element)  "<Heading>"
  Signal2ArrayOfSignals6/1(ArrayofElements) -> Activate_Switch/2(Heading)
  Bus Selector/5 -> Signal2ArrayOfSignals5/2(Element)  "<Velocity>"
  Signal2ArrayOfSignals5/1(ArrayofElements) -> Velocity [m/s]/1
  Bus Selector/4 -> Signal2ArrayOfSignals4/2(Element)  "<ID>"
  Signal2ArrayOfSignals4/1(ArrayofElements) -> Data Type Conversion/1, Activate_Switch/1(BeamID)
  Bus Selector/3 -> Signal2ArrayOfSignals3/2(Element)  "<Elevation>"
  Signal2ArrayOfSignals3/1(ArrayofElements) -> Elevation [deg]/1
  Bus Selector/2 -> Signal2ArrayOfSignals1/2(Element)  "<Azimuth>"
  Signal2ArrayOfSignals1/1(ArrayofElements) -> Azimuth [deg]/1
  Signal2ArrayOfSignals2/1(ArrayofElements) -> Range [m]/1
  Bus Selector/1 -> Signal2ArrayOfSignals2/2(Element)  "<Range>"
  Selector/1 -> Bus Selector/1
  For Iterator/1 -> Signal2ArrayOfSignals6/1(LoopIndex), Signal2ArrayOfSignals5/1(LoopIndex), Signal2ArrayOfSignals4/1(LoopIndex), Signal2ArrayOfSignals3/1(LoopIndex), Signal2ArrayOfSignals1/1(LoopIndex), Signal2ArrayOfSignals2/1(LoopIndex), Selector/2
  AIR/1 -> Selector/1
  Activate_Switch/1(On/Off) -> Heading [deg]/1

== system Base_Map_cs/Citroen_C3_Hatchback_1/Car_Pos_and_Orient ==
  In1 : Inport
  In2 : Inport  Port=2
  In3 : Inport  Port=3
  In4 : Inport  Port=4
  In5 : Inport  Port=5
  In6 : Inport  Port=6
  Data Type Conversion : DataTypeConversion
  Data Type Conversion1 : DataTypeConversion
  Data Type Conversion2 : DataTypeConversion
  Degrees to Radians1 : simulink_extras/Transformations/Degrees to Radians
  Degrees to Radians2 : simulink_extras/Transformations/Degrees to Radians
  Degrees to Radians5 : simulink_extras/Transformations/Degrees to Radians
  Mux : Mux
  Rotation Angles to Quaternions : sharedtransform/Rotation Angles to Quaternions  rotationOrder=XYZ  aMode=aMode
      settings: SourceProductName=Aerospace Blockset  SourceProductBaseCode=AE
  Vector Concatenate2 : Concatenate  NumInputs=3
  Out1 : Outport
  wires:
  Degrees to Radians1/1 -> Vector Concatenate2/2
  Degrees to Radians5/1 -> Vector Concatenate2/1
  Vector Concatenate2/1 -> Rotation Angles to Quaternions/1
  Degrees to Radians2/1 -> Vector Concatenate2/3
  In1/1 -> Data Type Conversion/1
  In2/1 -> Data Type Conversion1/1
  In3/1 -> Data Type Conversion2/1
  In4/1 -> Degrees to Radians5/1
  In5/1 -> Degrees to Radians1/1
  In6/1 -> Degrees to Radians2/1
  Data Type Conversion/1 -> Mux/1
  Data Type Conversion1/1 -> Mux/2
  Data Type Conversion2/1 -> Mux/3
  Rotation Angles to Quaternions/1 -> Mux/4
  Mux/1 -> Out1/1

== system Base_Map_cs/Citroen_C3_Hatchback_1/Dynamics_Empty ==
  note: For state mode 'Dynamic' positions
      | are not taken into account, as they
      | are computed by integrating velocity.
      | Click annotation for Help.
  Ground_{1..8} (8 alike) : Ground
  MuxState : Subsystem  Tag=mux/State  mask(Empty Dynamics State Block){positioningmode=on, TimeStep=1/300}
      mask prompts: positioningmode "Positioning Mode"; TimeStep "Auto Assigned: Time Step [s]"
      mask help:
      | Build the state of an actor based on user input.
      | The user can either use positioning mode or dynamics mode.
      | - When using positioning mode the position and orientation of the actor are set directly based on the input. Expected input is relative to the initial position and orientation of the actor. It's also possible to specify the velocity of the actor, though this input isn't used, only passed on.
      | - When using dynamics mode the position input is ignored. Expected input is velocity and orientation. The velocity is relative the current orientation of the actor, while orientation is relative to its initial orientation. The position of the actor is calculated based on the velocity and orientation given.
      settings: DeleteFcn=PreScanBlockDeleteFcn;
  STATE_Citroen_C3_Hatchback_1 : Subsystem  Tag=mux/StatePort  Priority=0  LoadFcn=load PrescanStateActuatorData  mask(PreScan Sink Block: State){x0=181.3426, y0=102.1129, z0=0.58, Roll0=0, Pitch0=0, Yaw0=0, TimeStep=1/300}
      mask prompts: x0 "Ini x-position VEHICLE wrt GLOBAL axis system [m]"; y0 "Ini y-position VEHICLE wrt GLOBAL axis system [m]"; z0 "Ini z-position VEHICLE wrt GLOBAL axis system [m]"; Roll0 "Ini roll-angle BODY wrt VEHICLE axis system [deg]"; Pitch0 "Ini pitch-angle BODY wrt VEHICLE axis system [deg]"; Yaw0 "Ini yaw-angle VEHICLE wrt GLOBAL axis system [deg]"; TimeStep "Auto-Assigned: Upload Period [s]"
      mask help:
      | The Actor State contains a vector signal of size (9x1), containing the following signals:
      |
      | -  Position                  (x,y,z)                                     [m]
      | -  Velocity                  (vx,vy,vz)                               [m/s]
      | -  Angles                    (Roll, Pitch, Yaw)                   [rad]
      |
      | The Actor state is defined in the global axis system.
      | The state is superponed on the Initial position defined in the GUI.
      |
      | For more information, please click Help.
      settings: DeleteFcn=PreScanBlockDeleteFcn;
      mask Help: eval('openHelp(222)')
      mask Display: image(imread('State.png'))
  Sine Wave Function : Sin  Amplitude=10  SampleTime=0
  State : Outport  Tag=outport/StateOutport  SampleTime=1/300
  wires:
  Sine Wave Function/1 -> MuxState/1(x [m])
  MuxState/1(state) -> STATE_Citroen_C3_Hatchback_1/1(State)
  STATE_Citroen_C3_Hatchback_1/1(StateBus) -> State/1
  Ground_1/1 -> MuxState/2(y [m])
  Ground_2/1 -> MuxState/3(z [m])
  Ground_3/1 -> MuxState/4(dx [m/s])
  Ground_4/1 -> MuxState/5(dy [m/s])
  Ground_5/1 -> MuxState/6(dz [m/s])
  Ground_6/1 -> MuxState/7(R [rad])
  Ground_7/1 -> MuxState/8(P [rad])
  Ground_8/1 -> MuxState/9(Y [rad])

== system Base_Map_cs/Citroen_C3_Hatchback_1/SELF_Demux ==
  SELF : Inport  OutDataTypeStr=Bus: PRESCAN_SELFSENSORDATA
  Bus Selector : BusSelector  OutputSignals=PositionX,PositionY,PositionZ,OrientationRoll,OrientationPitch,OrientationYaw,Velocity,Yaw_rate,Lat,Long,Alt
  Demux2 : Demux  Outputs=3
  Gain : Gain  Gain=180/pi
  Gain1 : Gain  Gain=180/pi
  Vector Concatenate1 : Concatenate  NumInputs=3
  compas converter : Subsystem
  x [m] : Outport
  y [m] : Outport  Port=2
  z [m] : Outport  Port=3
  rotx [deg] : Outport  Port=4
  roty [deg] : Outport  Port=5
  rotz [deg] : Outport  Port=6
  GPS lat [deg] : Outport  Port=7
  GPS long [deg] : Outport  Port=8
  GPS alt [m] : Outport  Port=9
  velocity [m/s] : Outport  Port=10
  heading [deg] : Outport  Port=11
  yaw rate [deg/s] : Outport  Port=12
  wires:
  Bus Selector/11 -> GPS alt [m]/1  "<Alt>"
  Bus Selector/10 -> GPS long [deg]/1  "<Long>"
  Bus Selector/9 -> GPS lat [deg]/1  "<Lat>"
  Bus Selector/8 -> Gain1/1  "<Yaw_rate>"
  Bus Selector/7 -> velocity [m/s]/1  "<Velocity>"
  Bus Selector/6 -> compas converter/1(rotz [rad]), Vector Concatenate1/3  "<OrientationYaw>"
  Bus Selector/5 -> Vector Concatenate1/2  "<OrientationPitch>"
  Bus Selector/4 -> Vector Concatenate1/1  "<OrientationRoll>"
  Vector Concatenate1/1 -> Gain/1
  Bus Selector/3 -> z [m]/1  "<PositionZ>"
  Bus Selector/2 -> y [m]/1  "<PositionY>"
  Bus Selector/1 -> x [m]/1  "<PositionX>"
  SELF/1 -> Bus Selector/1
  Gain/1 -> Demux2/1
  Demux2/1 -> rotx [deg]/1
  Demux2/2 -> roty [deg]/1
  Demux2/3 -> rotz [deg]/1
  compas converter/1(heading [deg]) -> heading [deg]/1
  Gain1/1 -> yaw rate [deg/s]/1

== system Base_Map_cs/Citroen_C3_Hatchback_1/message_creator ==
  In1 : Inport
  Blank Message4 : robotlib/Blank Message  messageClass=Message  entityType=geometry_msgs/Pose  messageType=geometry_msgs/Pose  SampleTime=inf
      settings: SourceProductBaseCode=RO
  Bus Assignment3 : BusAssignment  AssignedSignals=Position.X,Position.Y,Position.Z,Orientation.W,Orientation.X,Orientation.Y,Orientation.Z
  Demux : Demux  Outputs=7
  Out1 : Outport
  wires:
  Blank Message4/1 -> Bus Assignment3/1
  Demux/4 -> Bus Assignment3/5
  Demux/3 -> Bus Assignment3/4
  Demux/5 -> Bus Assignment3/6
  Demux/7 -> Bus Assignment3/8
  Demux/2 -> Bus Assignment3/3
  In1/1 -> Demux/1
  Demux/6 -> Bus Assignment3/7
  Demux/1 -> Bus Assignment3/2
  Bus Assignment3/1 -> Out1/1
